simulink model "multichannel_creater"  (R2017b)
settings: Solver=FixedStepDiscrete  StartTime=0.0  StopTime=60  RelTol=1e-3  EnableMultiTasking=on
model workspace (MAT data in the model file):
  h : matlab.ui.Figure (value not decoded)
  heli = [0 -3.0517578125e-05 -0.0001220703125 -0.000244140625 -0.0003662109375 -0.000701904296875 -0.00106811523438 -0.00204467773438 -0.00341796875 -0.00460815429688 -0.00595092773438 -0.00762939453125 ... (263304 elements, 263304x1)]
libraries: dspvision x4, dspindex x2
(part 1 of 2)
CloseFcn:
  | try
  |     h = evalin(get_param(gcs, 'ModelWorkspace'), 'h');
  |     close(h);
  | catch
  | end
settings Model: Creator=The MathWorks, Inc.  LastModifiedBy=13z
settings DataIOCC: LimitDataPoints=on  SaveFormat=Array
settings OptimizationCC: ExpressionDepthLimit=2147483647  RollThreshold=1  InitFltsAndDblsToZero=on  EfficientMapNaN2IntZero=off  LifeSpan=inf
settings DebuggingCC: UnderspecifiedInitializationDetection=Classic  MergeDetectMultiDrivingBlocksExec=none  InheritedTsInSrcMsg=none  FcnCallInpInsideContextMsg=warning  AllowSymbolicDim=off  StateNameClashWarn=warning  SFUnexpectedBacktrackingDiag=warning  SFNoUnconditionalDefaultTransitionDiag=warning  SFExecutionAtInitializationDiag=none
settings HardwareCC: ProdBitPerPointer=32  ProdBitPerSizeT=32  ProdBitPerPtrDiffT=32  ProdLargestAtomicFloat=None  ProdIntDivRoundTo=Undefined  ProdEndianess=Unspecified  ProdWordSize=32  ProdHWDeviceType=32-bit Generic
settings ModelReferenceCC: PropagateSignalLabelsOutOfModel=off
settings SFSimCC: SimParseCustomCode=off
settings CodeAppCC: StateflowObjectComments=on
settings GRTTargetCC: TargetLangStandard=C89/C90 (ANSI)  GeneratePreprocessorConditionals=Disable all  CombineOutputUpdateFcns=off  GRTInterface=on
settings ConfigComp: CovMetricSettings=dw  CovHtmlReporting=on  CovSaveCumulativeToWorkspaceVar=on  CovSaveSingleToWorkspaceVar=on  CovExternalEMLEnable=off  CovSFcnEnable=off

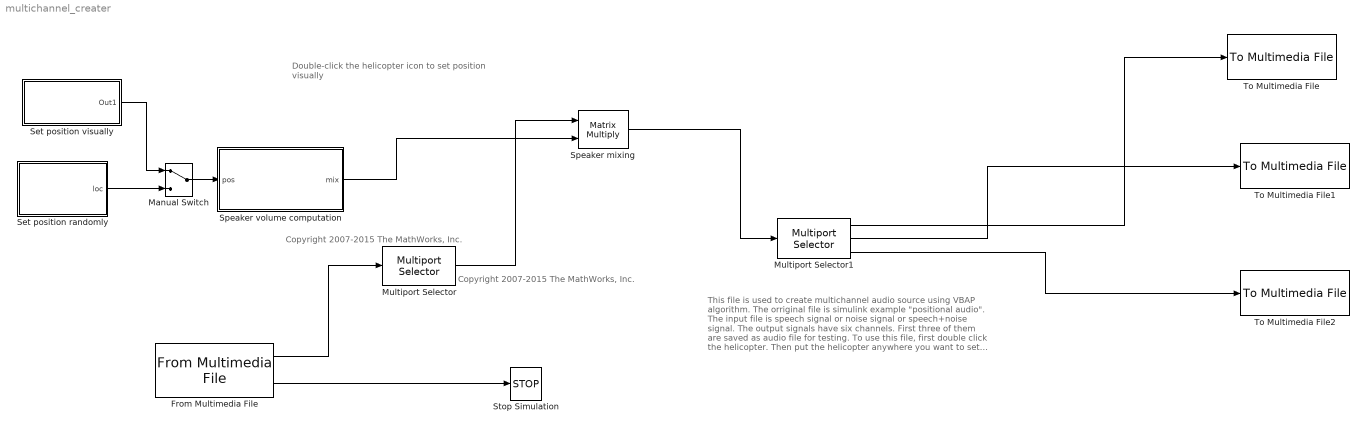
== system multichannel_creater ==
  note: This file is used to create multichannel audio source using VBAP algorithm. The orriginal file is simulink example "positional audio".
      |
      | The input file is speech signal or noise signal or speech+noise signal.
      |
      | The output signals have six channels. First three of them are saved as audio file for testing.
      |
      | To use this file, first double click the helicopter. Then put the helicopter anywhere you want to set visual position. And then run the block.
      |
      | More information refered to:
      | https://nl.mathworks.com/help/audio/examples/positional-audio.html
  note: Double-click the helicopter icon
      | to set position visually
  note: Copyright 2007-2015 The MathWorks, Inc.
  note: Copyright 2007-2015 The MathWorks, Inc.
  " Set position visually" : Subsystem  mask{loc=[0.1275 0.5925]}
      mask init:
      | I = imread('helicopter.jpg');
      settings: OpenFcn=assignin(get_param(gcs, 'ModelWorkspace'), 'h', HelperPositionalAudioUI(str2num(get_param(gcb,'loc')), gcb, @(blk,loc)(set_param(blk,'loc',loc))));
      mask Display: image(I);
  From Multimedia File : dspvision/From Multimedia File  inputFilename=D:\MATLAB\RD signal project\final_presentation\test environment\noise_7dB.wav  loop=on  numPlays=1  outputStreams=Audio only  videoDataType=single  audioDataType=double  inheritSampleTime=on  userDefinedSampleTime=1/30  noAudioOutput=off  isIntensityVideo=off  fourcc=RGB  colorVideoFormat=Separate color signals  outputEOF=on  dataOrg=Column-major  audioFrameSize=1024  computeAudioFrameSize=off  outSamplingMode=Sample based
      settings: SourceProductBaseCode=VP
  Manual Switch : ManualSwitch
  Multiport Selector : dspindex/Multiport Selector  rowsOrCols=Columns  idxCellArray={ 1 }  idxErrMode=Clip Index
  Multiport Selector1 : dspindex/Multiport Selector  rowsOrCols=Columns  idxCellArray={ 1 2 3 }  idxErrMode=Clip Index
  Set position randomly : MATLAB Function  TreatAsAtomicUnit=on
  Speaker mixing : Product  Multiplication=Matrix(*)
  Speaker volume computation : MATLAB Function  TreatAsAtomicUnit=on
  Stop Simulation : Stop
  To Multimedia File : dspvision/To Multimedia File  outputFilename=noise7dB_channel1.wav  streamSelection=Audio only  videoCompressor=None (uncompressed)  audioCompressor=None (uncompressed)  imagePorts=Separate color signals  fileType=WAV  audioDatatype=16-bit integer  fourcc=RGB  videoQuality=75  mj2000CompFactor=10
      settings: SourceProductName=Computer Vision System Toolbox  SourceProductBaseCode=VP
  To Multimedia File1 : dspvision/To Multimedia File  outputFilename=noise7dB_channel2.wav  streamSelection=Audio only  videoCompressor=None (uncompressed)  audioCompressor=None (uncompressed)  imagePorts=Separate color signals  fileType=WAV  audioDatatype=16-bit integer  fourcc=RGB  videoQuality=75  mj2000CompFactor=10
      settings: SourceProductName=Computer Vision System Toolbox  SourceProductBaseCode=VP
  To Multimedia File2 : dspvision/To Multimedia File  outputFilename=noise7dB_channel3.wav  streamSelection=Audio only  videoCompressor=None (uncompressed)  audioCompressor=None (uncompressed)  imagePorts=Separate color signals  fileType=WAV  audioDatatype=16-bit integer  fourcc=RGB  videoQuality=75  mj2000CompFactor=10
      settings: SourceProductName=Computer Vision System Toolbox  SourceProductBaseCode=VP
  wires:
  Speaker mixing/1 -> Multiport Selector1/1
  Multiport Selector1/1 -> To Multimedia File/1
  Multiport Selector1/2 -> To Multimedia File1/1
  Multiport Selector1/3 -> To Multimedia File2/1
  Set position randomly/1(loc) -> Manual Switch/2
  " Set position visually"/1(Out1) -> Manual Switch/1
  Manual Switch/1 -> Speaker volume computation/1(pos)
  Speaker volume computation/1(mix) -> Speaker mixing/2
  From Multimedia File/2 -> Stop Simulation/1
  From Multimedia File/1 -> Multiport Selector/1
  Multiport Selector/1 -> Speaker mixing/1
